simulink model "project7420"  (Simulink 7.8)
settings: Solver=ode45  StartTime=0.0  StopTime=50  RelTol=1e-3
settings Model: Creator=CC  LastModifiedBy=CC

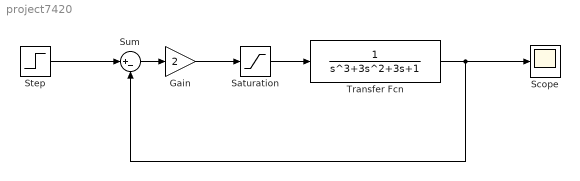
== system project7420 ==
  Gain : Gain  Gain=2
  Saturation : Saturate
  Scope : Scope
      settings: YMin=0  YMax=1.1  SaveName=ScopeData2
  Step : Step  Before=2  SampleTime=0
  Sum : Sum  Inputs=|+-
  Transfer Fcn : TransferFcn  Denominator=[1 3 3 1]
  wires:
  Transfer Fcn/1 -> Scope/1, Sum/2
  Step/1 -> Sum/1
  Sum/1 -> Gain/1
  Gain/1 -> Saturation/1
  Saturation/1 -> Transfer Fcn/1
